simulink model "slave_site"  (R2019a)
settings: Solver=FixedStepAuto  StartTime=0.0  StopTime=inf  FixedStep=0.001  RelTol=1e-3
libraries: dspnetwork x16, etargetslib x1
settings Model: SimulationMode=accelerator  EnablePacing=on  Creator=jakub  LastModifiedBy=kirill
settings SolverCC: AutoInsertRateTranBlk=on
settings DataIOCC: ReturnWorkspaceOutputs=off
settings HardwareCC: ProdBitPerLong=64  ProdHWDeviceType=Intel->x86-64 (Linux 64)

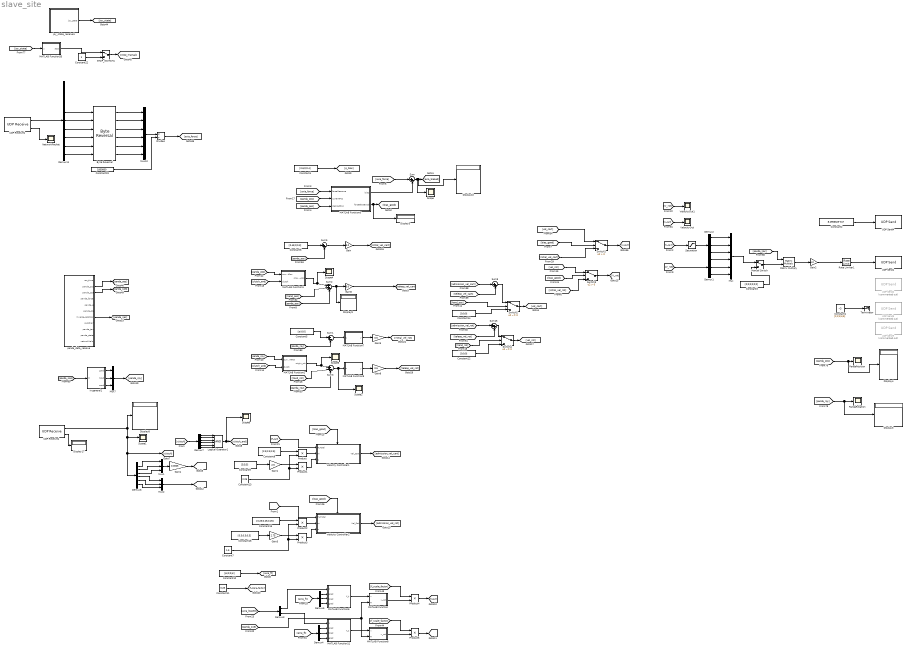
== system slave_site ==
  Byte Reversal : etargetslib/Byte Reversal  numInp=6
      settings: SourceProductName=MATLAB Coder  SourceProductBaseCode=ME
  Constant1 : Constant  Value=[1;2;3;4;5]  OutDataTypeStr=double
  Constant10 : Constant  Value=[pi/2;0;pi]
  Constant11 : Constant  Value=0.25
  Constant12 : Constant  Value=[0;0;0]
  Constant13 : Constant  Value=2.25
  Constant14 : Constant  Value=[0;0;0]
  Constant15 : Constant  Value=[0.25;0.25;0.25]
  Constant16 : Constant  Value=[0.5;0.5;0.5]
  Constant2 : Constant  Value=8.295632e-317  OutDataTypeStr=double
  Constant22 : Constant
  Constant23 : Constant  Value=1000000
  Constant3 : Constant  Value=[0;0;0;0;0;0]
  Constant4 : Constant  Value=[0.6;0;0.4]
  Constant5 : Constant  Value=[pi;0;0]
  Constant6 : Constant  Value=[0.45;0;0.3]
  Constant7 : Constant  Value=1.5
  Constant8 : Constant  Value=[2.5;2.5;2.5]
  Constant9 : Constant  Value=[5;5;5]
  Demux{1..2,4..5} (4 alike) : Demux  Outputs=3
  Demux11 : Demux  Outputs=9
  Demux3 : Demux  Outputs=2
  Demux6 : Demux  Outputs=6
  Demux7 : Demux  Outputs=6
  Display{3..5,8..10,17} (7 alike) : Display
      Display3 settings: Decimation=4
      Display4 settings: Decimation=4
  Divide4 : Product  Inputs=*/  OutDataTypeStr=double
  Gain : Gain  Gain=3.0
  Gain1 : Gain  Gain=2.5
  Gain2 : Gain  Gain=1.0
  Gain3 : Gain  Gain=2.75
  Gain4 : Gain  Gain=0.0005
  Gain5 : Gain  Gain=0.5
  Gain6 : Gain  Gain=3.0
  Gain8 : Gain  Gain=0.5
  Logical Operator1 : Logic  Inputs=6  AllPortsSameDT=off  OutDataTypeStr=boolean
  MATLAB Function : MATLAB Function  TreatAsAtomicUnit=on
  MATLAB Function1 : MATLAB Function  TreatAsAtomicUnit=on
  MATLAB Function11 : MATLAB Function  TreatAsAtomicUnit=on
  MATLAB Function2 : MATLAB Function  TreatAsAtomicUnit=on
  MATLAB Function33 : MATLAB Function  TreatAsAtomicUnit=on
  MATLAB Function5 : MATLAB Function  TreatAsAtomicUnit=on
  MATLAB Function6 : MATLAB Function  TreatAsAtomicUnit=on
  MATLAB Function7 : MATLAB Function  TreatAsAtomicUnit=on
  MATLAB Function8 : MATLAB Function  TreatAsAtomicUnit=on
  MATLAB Function9 : MATLAB Function  TreatAsAtomicUnit=on
  Manual Switch : ManualSwitch
  Matrix Multiply : Product  Multiplication=Matrix(*)
  Mux : Mux  Inputs=6
  Mux1 : Mux  Inputs=3
  Mux10 : Mux  Inputs=6
  Mux2 : Mux  Inputs=3
  Mux7 : Mux  Inputs=3
  NetworkPacket : Scope
  PandaPosition : Scope
  PandaRotation : Scope
  Product{,1..5} (6 alike) : Product
  Rate Limiter1 : RateLimiter  RisingSlewLimit=2.0  FallingSlewLimit=-2.0  SampleTimeMode=inherited
  STOP_SWITCH1 : ManualSwitch
  Saturation : Saturate  UpperLimit=0.1  LowerLimit=-0.1
  Scope{,1..2,4..6} (6 alike) : Scope
  Sum : Sum  Inputs=|+-
  Sum1 : Sum  Inputs=|+-
  Sum15 : Sum  Inputs=|++
  Sum2 : Sum  Inputs=|++-
  Sum3 : Sum  Inputs=|++-
  Sum5 : Sum  Inputs=|+-
  Sum9 : Sum  Inputs=|++
  Switch1 : Switch  Criteria=u2 > Threshold
  Switch2 : Switch  Criteria=u2 ~= 0
  Switch3 : Switch  Criteria=u2 > Threshold
  Switch4 : Switch  Criteria=u2 ~= 0
  Terminator : Terminator
  UDP Receive1 : dspnetwork/UDP Receive  localURL='0.0.0.0'  localPort=49154  remoteURL='192.168.0.13'  remotePort=-1  recvBufferSize=36  dims=9  signalDatatype=int32  isComplex=off  isVarSize=off  showBlockingTime=off  blockingTime=0  sampletime=0.001  blockPlatform=[]
      settings: SourceProductName=Simulink
  UDP Receive4 : dspnetwork/UDP Receive  localURL='0.0.0.0'  localPort=8005  remoteURL='192.168.0.110'  remotePort=-1  recvBufferSize=12288  dims=6  signalDatatype=double  isComplex=off  isVarSize=off  showBlockingTime=off  blockingTime=0  sampletime=0.001  blockPlatform=[]
      settings: SourceProductName=Simulink
  UDP Send1 : dspnetwork/UDP Send  remoteURL='127.0.0.1'  remotePort=39474  localURL='0.0.0.0'  localPortSource=Automatically determine  localPort=48000  sampletime=-1  blockPlatform=[]  separateLengthPort=0
      settings: SourceProductName=Simulink
  UDP Send2 : dspnetwork/UDP Send  Commented=on  remoteURL='255.255.255.255'  remotePort=39474  localURL='0.0.0.0'  localPortSource=Automatically determine  localPort=-1  sampletime=-1  blockPlatform=[]  separateLengthPort=0
      settings: SourceProductName=Simulink
  UDP Send3 : dspnetwork/UDP Send  Commented=on  remoteURL='192.168.0.20'  remotePort=40001  localURL='0.0.0.0'  localPortSource=Specify via dialog  localPort=49001  sampletime=-1  blockPlatform=[]  separateLengthPort=0
      settings: SourceProductName=Simulink
  UDP Send4 : dspnetwork/UDP Send  remoteURL='192.168.0.13'  remotePort=49152  localURL='0.0.0.0'  localPortSource=Specify via dialog  localPort=49154  sampletime=-1  blockPlatform=[]  separateLengthPort=0
      settings: SourceProductName=Simulink
  UDP Send5 : dspnetwork/UDP Send  Commented=on  remoteURL='127.0.0.1'  remotePort=40001  localURL='0.0.0.0'  localPortSource=Specify via dialog  localPort=49001  sampletime=-1  blockPlatform=[]  separateLengthPort=0
      settings: SourceProductName=Simulink
  Velocity Controller1 : Subsystem
  Velocity Controller2 : Subsystem
  VelocityOut : Scope
  VelocityOut1 : Scope
  in general1 : MATLAB Function  TreatAsAtomicUnit=on
  joy_state_receive1 : Subsystem
  panda_data_receive : Subsystem
  wires:
  Demux2/1 -> Mux/1
  Demux1/2 -> Mux/5
  Demux1/1 -> Mux/4
  Demux2/2 -> Mux/2
  Demux1/3 -> Mux/6
  Demux2/3 -> Mux/3
  joy_state_receive1/1("joy_state ") -> [joy_state]
  [joy_state] -> MATLAB Function33/1(u)
  MATLAB Function33/1(stop) -> STOP_SWITCH1/1
  STOP_SWITCH1/1 -> [stop_manual]
  Constant22/1 -> STOP_SWITCH1/2
  [panda_so3] -> in general1/1(R)
  in general1/2(brad) -> Mux7/2
  Mux7/1 -> [panda_rpy]
  [panda_ijac] -> Matrix Multiply/1
  UDP Receive1/2 -> NetworkPacket/1
  Byte Reversal/4 -> Mux10/4
  Divide4/1 -> [axia_force]
  Byte Reversal/2 -> Mux10/2
  Constant23/1 -> Divide4/2
  Demux11/7 -> Byte Reversal/4
  Mux10/1 -> Divide4/1
  Byte Reversal/1 -> Mux10/1
  Demux11/5 -> Byte Reversal/2
  UDP Receive1/1 -> Demux11/1
  Demux11/6 -> Byte Reversal/3
  Byte Reversal/3 -> Mux10/3
  Demux11/9 -> Byte Reversal/6
  Demux11/8 -> Byte Reversal/5
  Demux11/4 -> Byte Reversal/1
  Byte Reversal/5 -> Mux10/5
  Byte Reversal/6 -> Mux10/6
  [panda_pos] -> Display4/1, PandaPosition/1
  [V_cart] -> VelocityOut/1
  panda_data_receive/2(panda_pos) -> [panda_pos]
  panda_data_receive/3(panda_so3) -> [panda_so3]
  panda_data_receive/7(inverse_jacobian) -> [panda_ijac]
  [panda_rpy] -> Display3/1, PandaRotation/1
  [panda_rpy] -> Sum1/2
  Gain2/1 -> Rate Limiter1/1
  Matrix Multiply/1 -> Gain2/1
  Constant2/1 -> UDP Send4/1
  Constant1/1 -> Terminator/1
  Sum5/1 -> Gain/1
  [panda_pos] -> Sum5/2
  Saturation/1 -> Demux2/1
  Mux/1 -> Manual Switch/1
  Manual Switch/1 -> Matrix Multiply/2
  Constant3/1 -> Manual Switch/2
  MATLAB Function5/1(bias) -> Sum/2
  [axia_force] -> Sum/1
  Sum/1 -> Scope/1, Display10/1, [axia_biased]
  Sum1/1 -> MATLAB Function7/1(u)
  MATLAB Function7/1(y) -> Gain5/1
  MATLAB Function5/2(forceBiasGood) -> Display5/1, [bias_good]
  Constant4/1 -> [p_bias]
  [axia_force] -> MATLAB Function5/1(forceMeasure)
  [panda_pos] -> MATLAB Function5/2(currentPos)
  [panda_pos] -> MATLAB Function5/3(desiredPos)
  Constant11/1 -> [f_scale_factor]
  MATLAB Function8/1(x_rot) -> Product5/2
  MATLAB Function/1(x_rot) -> Product4/2
  Demux3/2 -> MATLAB Function11/1(X)
  Demux4/2 -> MATLAB Function11/3(brad)
  Demux5/3 -> MATLAB Function6/4(grad)
  Demux3/1 -> MATLAB Function6/1(X)
  [axia_ft] -> Demux5/1
  Demux4/3 -> MATLAB Function11/4(grad)
  Demux4/1 -> MATLAB Function11/2(arad)
  [axia_ft] -> Demux4/1
  MATLAB Function6/1(X_t) -> MATLAB Function/1(x)
  [f_scale_factor] -> Product5/1
  [f_scale_factor] -> Product4/1
  Product4/1 -> [F_cart]
  MATLAB Function11/1(X_t) -> MATLAB Function8/1(x)
  [panda_so3] -> MATLAB Function/2(R), MATLAB Function8/2(R)
  Demux5/2 -> MATLAB Function6/3(brad)
  Product5/1 -> [M_cart]
  Gain1/1 -> Product1/1
  Constant8/1 -> Product/1
  Constant9/1 -> Gain1/1
  Product/1 -> Velocity Controller1/2(m)
  Product1/1 -> Velocity Controller1/3(c)
  [F_cart] -> Velocity Controller1/1(F_Total)
  Switch1/1 -> [V_cart]
  Demux5/1 -> MATLAB Function6/2(arad)
  Constant13/1 -> Product1/2, Product/2
  [V_rot] -> VelocityOut1/1
  [axia_biased] -> Demux3/1
  Gain3/1 -> Product3/1
  Product3/1 -> Velocity Controller2/3(c)
  Constant7/1 -> Product2/2, Product3/2
  Constant16/1 -> Gain3/1
  Product2/1 -> Velocity Controller2/2(m)
  Constant15/1 -> Product2/1
  [M_cart] -> Velocity Controller2/1(M_Total)
  Switch3/1 -> [V_rot]
  [bias_good] -> Velocity Controller1/Enable
  Gain5/1 -> [initial_vel_rot]
  [initial_vel_rot] -> Switch3/3
  [bias_good] -> Velocity Controller2/Enable
  Velocity Controller2/1(Vel_Rot) -> [admission_vel_rot]
  Velocity Controller1/1(Vel_Cart) -> [admission_vel_cart]
  Gain/1 -> [initial_vel_cart]
  [initial_vel_cart] -> Switch1/3
  [vel_rot] -> Switch3/1
  [hand_pos] -> Sum2/2
  [admission_vel_cart] -> Sum9/1
  [teleop_vel_cart] -> Sum9/2
  UDP Receive4/2 -> Display17/1
  Rate Limiter1/1 -> UDP Send1/1
  [teleop_vel_rot] -> Sum15/2
  [admission_vel_rot] -> Sum15/1
  MATLAB Function9/1(y) -> Gain8/1
  [panda_rpy] -> Sum3/3
  Sum3/1 -> Scope2/1, MATLAB Function9/1(u)
  [hand_rot] -> Sum3/2
  Gain8/1 -> [teleop_vel_rot]
  UDP Receive4/1 -> Display8/1, Scope1/1, Demux6/1, [clutch]
  [vel_cart] -> Switch1/1
  Constant6/1 -> Sum5/1
  Constant10/1 -> [axia_ft]
  in general1/3(arad) -> Mux7/3
  in general1/1(grad) -> Mux7/1
  [panda_pos] -> Sum2/3
  Sum2/1 -> Gain6/1, Display9/1
  Demux6/3 -> Mux1/3
  Demux6/2 -> Mux1/2
  Demux6/1 -> Mux1/1
  Mux1/1 -> Gain4/1
  Demux6/4 -> Mux2/1
  Demux6/5 -> Mux2/2
  Demux6/6 -> Mux2/3
  [bias_good] -> Switch1/2
  [panda_pos] -> MATLAB Function1/1(currentPos)
  MATLAB Function1/1(origin_pos) -> Scope4/1, Sum2/1
  [clutch_and] -> MATLAB Function1/2(clutch)
  Demux7/1 -> Logical Operator1/1
  Demux7/2 -> Logical Operator1/2
  Demux7/6 -> Logical Operator1/6
  Demux7/3 -> Logical Operator1/3
  Demux7/4 -> Logical Operator1/4
  [clutch] -> Demux7/1
  Demux7/5 -> Logical Operator1/5
  Logical Operator1/1 -> Scope6/1, [clutch_and]
  Gain4/1 -> [hand_pos]
  Mux2/1 -> [hand_rot]
  Constant5/1 -> Sum1/1
  [bias_good] -> Switch3/2
  [clutch_and] -> MATLAB Function2/2(clutch)
  [panda_rpy] -> MATLAB Function2/1(currentRot)
  MATLAB Function2/1(origin_rot) -> Scope5/1, Sum3/1
  Switch2/1 -> [vel_cart]
  Sum9/1 -> Switch2/1
  Constant14/1 -> Switch2/3
  [hand_pos] -> Switch2/2
  Switch4/1 -> [vel_rot]
  Sum15/1 -> Switch4/1
  Constant12/1 -> Switch4/3
  [hand_rot] -> Switch4/2
  Gain6/1 -> [teleop_vel_cart]
  [V_cart] -> Saturation/1
  [V_rot] -> Demux1/1

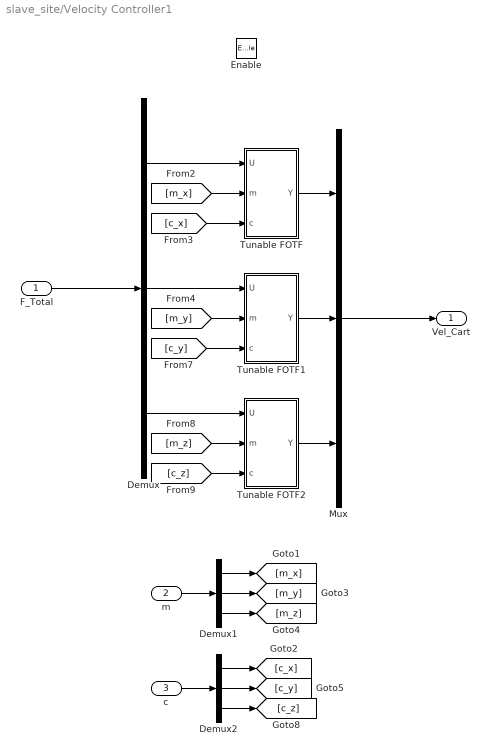
== system slave_site/Velocity Controller1 ==
  F_Total : Inport
  m : Inport  Port=2
  c : Inport  Port=3
  Enable : EnablePort
  Demux : Demux  Outputs=3
  Demux1 : Demux  Outputs=3
  Demux2 : Demux  Outputs=3
  Mux : Mux  Inputs=3
  Tunable FOTF : Subsystem
  Tunable FOTF1 : Subsystem
  Tunable FOTF2 : Subsystem
  Vel_Cart : Outport
  wires:
  [m_y] -> Tunable FOTF1/2(m)
  [c_x] -> Tunable FOTF/3(c)
  Demux/1 -> Tunable FOTF/1(U)
  Tunable FOTF2/1(Y) -> Mux/3
  [m_z] -> Tunable FOTF2/2(m)
  Mux/1 -> Vel_Cart/1
  [c_y] -> Tunable FOTF1/3(c)
  [m_x] -> Tunable FOTF/2(m)
  [c_z] -> Tunable FOTF2/3(c)
  Tunable FOTF/1(Y) -> Mux/1
  Demux/2 -> Tunable FOTF1/1(U)
  F_Total/1 -> Demux/1
  Tunable FOTF1/1(Y) -> Mux/2
  Demux/3 -> Tunable FOTF2/1(U)
  Demux2/2 -> [c_y]
  Demux1/2 -> [m_y]
  c/1 -> Demux2/1
  m/1 -> Demux1/1
  Demux2/1 -> [c_x]
  Demux1/1 -> [m_x]
  Demux1/3 -> [m_z]
  Demux2/3 -> [c_z]

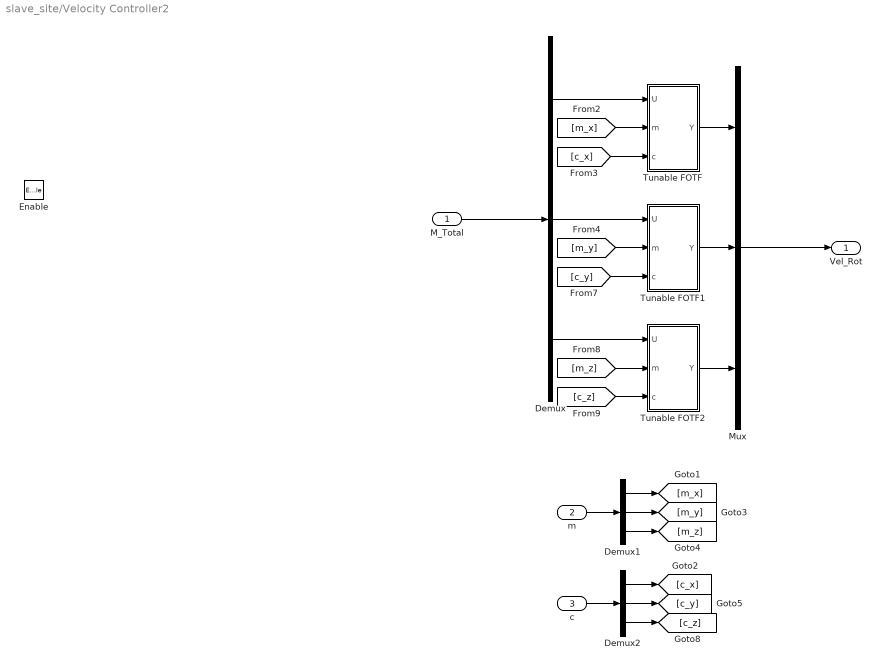
== system slave_site/Velocity Controller2 ==
  M_Total : Inport
  m : Inport  Port=2
  c : Inport  Port=3
  Enable : EnablePort
  Demux : Demux  Outputs=3
  Demux1 : Demux  Outputs=3
  Demux2 : Demux  Outputs=3
  Mux : Mux  Inputs=3
  Tunable FOTF : Subsystem
  Tunable FOTF1 : Subsystem
  Tunable FOTF2 : Subsystem
  Vel_Rot : Outport
  wires:
  [m_y] -> Tunable FOTF1/2(m)
  [c_x] -> Tunable FOTF/3(c)
  Demux/1 -> Tunable FOTF/1(U)
  Tunable FOTF2/1(Y) -> Mux/3
  [m_z] -> Tunable FOTF2/2(m)
  Mux/1 -> Vel_Rot/1
  [c_y] -> Tunable FOTF1/3(c)
  [m_x] -> Tunable FOTF/2(m)
  [c_z] -> Tunable FOTF2/3(c)
  Tunable FOTF/1(Y) -> Mux/1
  Demux/2 -> Tunable FOTF1/1(U)
  M_Total/1 -> Demux/1
  Tunable FOTF1/1(Y) -> Mux/2
  Demux/3 -> Tunable FOTF2/1(U)
  Demux2/2 -> [c_y]
  Demux1/2 -> [m_y]
  c/1 -> Demux2/1
  m/1 -> Demux1/1
  Demux2/1 -> [c_x]
  Demux1/1 -> [m_x]
  Demux1/3 -> [m_z]
  Demux2/3 -> [c_z]

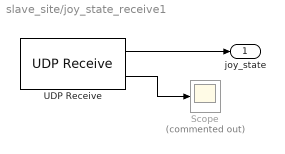
== system slave_site/joy_state_receive1 ==
  Scope : Scope  Commented=on
  UDP Receive : dspnetwork/UDP Receive  localURL='0.0.0.0'  localPort=33333  remoteURL='0.0.0.0'  remotePort=-1  recvBufferSize=840  dims=21  signalDatatype=single  isComplex=off  isVarSize=off  showBlockingTime=off  blockingTime=0  sampletime=0.001  blockPlatform=[]
      settings: SourceProductName=Simulink
  "joy_state " : Outport
  wires:
  UDP Receive/2 -> Scope/1
  UDP Receive/1 -> "joy_state "/1

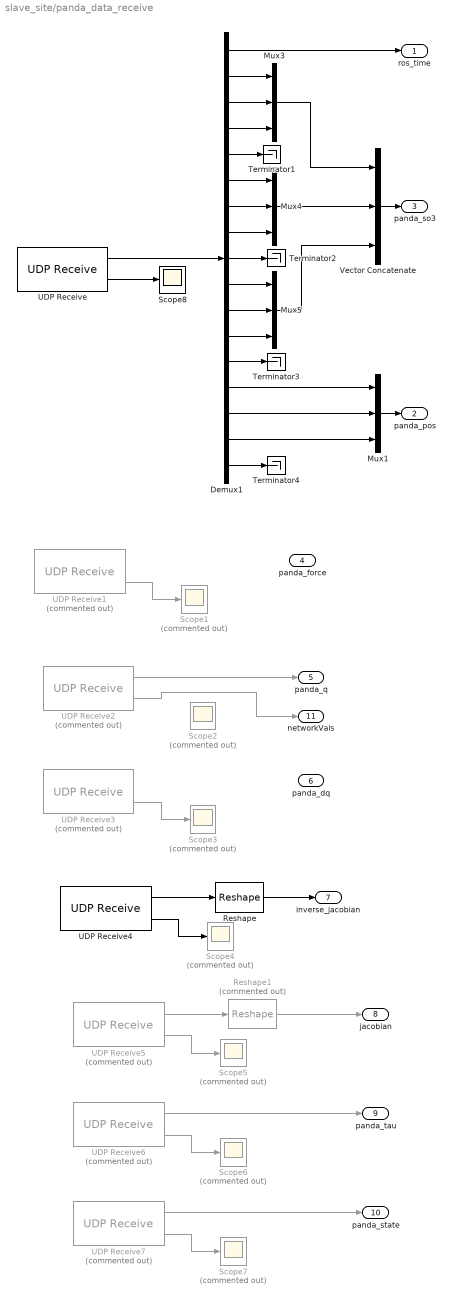
== system slave_site/panda_data_receive ==
  Demux1 : Demux  Outputs=17
  Mux{1,3..5} (4 alike) : Mux  Inputs=3
  Reshape : Reshape  OutputDimensionality=Customize  OutputDimensions=[7,6]
  Reshape1 : Reshape  Commented=on  OutputDimensionality=Customize  OutputDimensions=[7,6]
  Scope{1..7} (7 alike) : Scope  Commented=on
  Scope8 : Scope
  Terminator{1..4} (4 alike) : Terminator
  UDP Receive : dspnetwork/UDP Receive  localURL='0.0.0.0'  localPort=30001  remoteURL='127.0.0.1'  remotePort=-1  recvBufferSize=4096  dims=17  signalDatatype=double  isComplex=off  isVarSize=off  showBlockingTime=off  blockingTime=0  sampletime=0.001  blockPlatform=[]
      settings: SourceProductName=Simulink
  UDP Receive1 : dspnetwork/UDP Receive  Commented=on  localURL='0.0.0.0'  localPort=30002  remoteURL='0.0.0.0'  remotePort=-1  recvBufferSize=48  dims=6  signalDatatype=double  isComplex=off  isVarSize=off  showBlockingTime=off  blockingTime=0  sampletime=0.001  blockPlatform=[]
      settings: SourceProductName=Simulink
  UDP Receive2 : dspnetwork/UDP Receive  Commented=on  localURL='0.0.0.0'  localPort=30003  remoteURL='0.0.0.0'  remotePort=-1  recvBufferSize=56  dims=7  signalDatatype=double  isComplex=off  isVarSize=off  showBlockingTime=off  blockingTime=0  sampletime=0.001  blockPlatform=[]
      settings: SourceProductName=Simulink
  UDP Receive3 : dspnetwork/UDP Receive  Commented=on  localURL='0.0.0.0'  localPort=30004  remoteURL='0.0.0.0'  remotePort=-1  recvBufferSize=56  dims=7  signalDatatype=double  isComplex=off  isVarSize=off  showBlockingTime=off  blockingTime=0  sampletime=0.001  blockPlatform=[]
      settings: SourceProductName=Simulink
  UDP Receive4 : dspnetwork/UDP Receive  localURL='0.0.0.0'  localPort=30005  remoteURL='0.0.0.0'  remotePort=-1  recvBufferSize=3360  dims=42  signalDatatype=double  isComplex=off  isVarSize=off  showBlockingTime=off  blockingTime=0  sampletime=0.001  blockPlatform=[]
      settings: SourceProductName=Simulink
  UDP Receive5 : dspnetwork/UDP Receive  Commented=on  localURL='0.0.0.0'  localPort=30006  remoteURL='0.0.0.0'  remotePort=-1  recvBufferSize=3360  dims=42  signalDatatype=double  isComplex=off  isVarSize=off  showBlockingTime=off  blockingTime=0  sampletime=0.001  blockPlatform=[]
      settings: SourceProductName=Simulink
  UDP Receive6 : dspnetwork/UDP Receive  Commented=on  localURL='0.0.0.0'  localPort=30010  remoteURL='0.0.0.0'  remotePort=-1  recvBufferSize=56  dims=7  signalDatatype=double  isComplex=off  isVarSize=off  showBlockingTime=off  blockingTime=0  sampletime=0.001  blockPlatform=[]
      settings: SourceProductName=Simulink
  UDP Receive7 : dspnetwork/UDP Receive  Commented=on  localURL='0.0.0.0'  localPort=30030  remoteURL='0.0.0.0'  remotePort=-1  recvBufferSize=40  dims=1  signalDatatype=uint8  isComplex=off  isVarSize=off  showBlockingTime=off  blockingTime=0  sampletime=0.001  blockPlatform=[]
      settings: SourceProductName=Simulink
  Vector Concatenate : Concatenate  NumInputs=3  Mode=Multidimensional array  ConcatenateDimension=2
  ros_time : Outport
  panda_pos : Outport  Port=2
  panda_so3 : Outport  Port=3
  panda_force : Outport  Port=4
  panda_q : Outport  Port=5
  panda_dq : Outport  Port=6
  inverse_jacobian : Outport  Port=7
  jacobian : Outport  Port=8
  panda_tau : Outport  Port=9
  panda_state : Outport  Port=10
  networkVals : Outport  Port=11
  wires:
  Mux1/1 -> panda_pos/1
  Demux1/6 -> Mux4/1
  Mux3/1 -> Vector Concatenate/1
  Demux1/10 -> Mux5/1
  Demux1/7 -> Mux4/2
  Demux1/12 -> Mux5/3
  Demux1/16 -> Mux1/3
  Demux1/9 -> Terminator2/1
  Demux1/4 -> Mux3/3
  Demux1/15 -> Mux1/2
  Demux1/5 -> Terminator1/1
  Demux1/2 -> Mux3/1
  Demux1/3 -> Mux3/2
  Demux1/1 -> ros_time/1
  Demux1/14 -> Mux1/1
  Mux4/1 -> Vector Concatenate/2
  Demux1/8 -> Mux4/3
  Demux1/11 -> Mux5/2
  Vector Concatenate/1 -> panda_so3/1
  Demux1/13 -> Terminator3/1
  Demux1/17 -> Terminator4/1
  Mux5/1 -> Vector Concatenate/3
  UDP Receive1/2 -> Scope1/1
  UDP Receive2/1 -> panda_q/1
  UDP Receive3/2 -> Scope3/1
  Reshape/1 -> inverse_jacobian/1
  UDP Receive4/2 -> Scope4/1
  UDP Receive4/1 -> Reshape/1
  Reshape1/1 -> jacobian/1
  UDP Receive5/1 -> Reshape1/1
  UDP Receive5/2 -> Scope5/1
  UDP Receive6/1 -> panda_tau/1
  UDP Receive6/2 -> Scope6/1
  UDP Receive7/1 -> panda_state/1
  UDP Receive7/2 -> Scope7/1
  UDP Receive2/2 -> networkVals/1
  UDP Receive/2 -> Scope8/1
  UDP Receive/1 -> Demux1/1

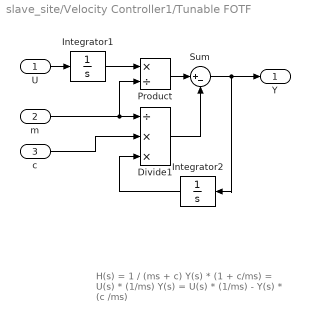
== system slave_site/Velocity Controller1/Tunable FOTF ==
  note: H(s) = 1 / (ms + c)
      | Y(s) * (1 + c/ms) = U(s) * (1/ms)
      | Y(s) = U(s) * (1/ms) - Y(s) * (c /ms)
  U : Inport
  m : Inport  Port=2
  c : Inport  Port=3
  Divide1 : Product  Inputs=/**
  Integrator1 : Integrator
  Integrator2 : Integrator
  Product : Product  Inputs=*/
  Sum : Sum  Inputs=|+-
  Y : Outport
  wires:
  U/1 -> Integrator1/1
  Integrator1/1 -> Product/1
  m/1 -> Divide1/1, Product/2
  Product/1 -> Sum/1
  Sum/1 -> Integrator2/1, Y/1
  c/1 -> Divide1/2
  Divide1/1 -> Sum/2
  Integrator2/1 -> Divide1/3

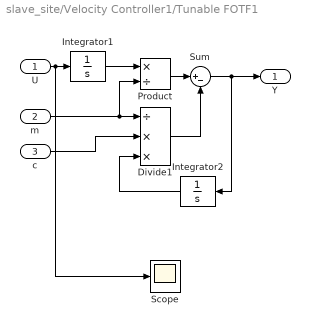
== system slave_site/Velocity Controller1/Tunable FOTF1 ==
  U : Inport
  m : Inport  Port=2
  c : Inport  Port=3
  Divide1 : Product  Inputs=/**
  Integrator1 : Integrator
  Integrator2 : Integrator
  Product : Product  Inputs=*/
  Scope : Scope
  Sum : Sum  Inputs=|+-
  Y : Outport
  wires:
  U/1 -> Scope/1, Integrator1/1
  Integrator1/1 -> Product/1
  m/1 -> Divide1/1, Product/2
  Product/1 -> Sum/1
  Sum/1 -> Integrator2/1, Y/1
  c/1 -> Divide1/2
  Divide1/1 -> Sum/2
  Integrator2/1 -> Divide1/3

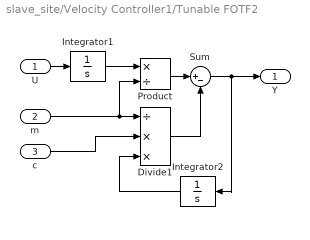
== system slave_site/Velocity Controller1/Tunable FOTF2 ==
  U : Inport
  m : Inport  Port=2
  c : Inport  Port=3
  Divide1 : Product  Inputs=/**
  Integrator1 : Integrator
  Integrator2 : Integrator
  Product : Product  Inputs=*/
  Sum : Sum  Inputs=|+-
  Y : Outport
  wires:
  U/1 -> Integrator1/1
  Integrator1/1 -> Product/1
  m/1 -> Divide1/1, Product/2
  Product/1 -> Sum/1
  Sum/1 -> Integrator2/1, Y/1
  c/1 -> Divide1/2
  Divide1/1 -> Sum/2
  Integrator2/1 -> Divide1/3

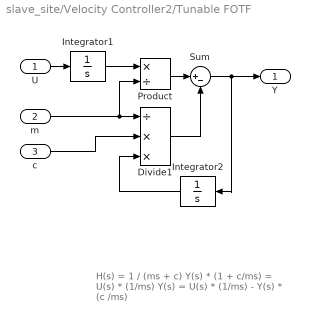
== system slave_site/Velocity Controller2/Tunable FOTF ==
  note: H(s) = 1 / (ms + c)
      | Y(s) * (1 + c/ms) = U(s) * (1/ms)
      | Y(s) = U(s) * (1/ms) - Y(s) * (c /ms)
  U : Inport
  m : Inport  Port=2
  c : Inport  Port=3
  Divide1 : Product  Inputs=/**
  Integrator1 : Integrator
  Integrator2 : Integrator
  Product : Product  Inputs=*/
  Sum : Sum  Inputs=|+-
  Y : Outport
  wires:
  U/1 -> Integrator1/1
  Integrator1/1 -> Product/1
  m/1 -> Divide1/1, Product/2
  Product/1 -> Sum/1
  Sum/1 -> Integrator2/1, Y/1
  c/1 -> Divide1/2
  Divide1/1 -> Sum/2
  Integrator2/1 -> Divide1/3

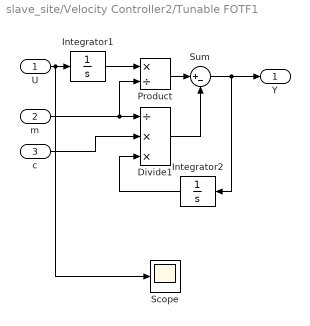
== system slave_site/Velocity Controller2/Tunable FOTF1 ==
  U : Inport
  m : Inport  Port=2
  c : Inport  Port=3
  Divide1 : Product  Inputs=/**
  Integrator1 : Integrator
  Integrator2 : Integrator
  Product : Product  Inputs=*/
  Scope : Scope
  Sum : Sum  Inputs=|+-
  Y : Outport
  wires:
  U/1 -> Scope/1, Integrator1/1
  Integrator1/1 -> Product/1
  m/1 -> Divide1/1, Product/2
  Product/1 -> Sum/1
  Sum/1 -> Integrator2/1, Y/1
  c/1 -> Divide1/2
  Divide1/1 -> Sum/2
  Integrator2/1 -> Divide1/3

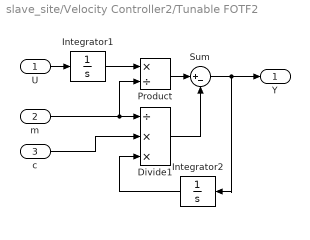
== system slave_site/Velocity Controller2/Tunable FOTF2 ==
  U : Inport
  m : Inport  Port=2
  c : Inport  Port=3
  Divide1 : Product  Inputs=/**
  Integrator1 : Integrator
  Integrator2 : Integrator
  Product : Product  Inputs=*/
  Sum : Sum  Inputs=|+-
  Y : Outport
  wires:
  U/1 -> Integrator1/1
  Integrator1/1 -> Product/1
  m/1 -> Divide1/1, Product/2
  Product/1 -> Sum/1
  Sum/1 -> Integrator2/1, Y/1
  c/1 -> Divide1/2
  Divide1/1 -> Sum/2
  Integrator2/1 -> Divide1/3

== matlab function slave_site/MATLAB Function2 ==
  data: currentRot input; origin_rot output; clutch input
function origin_rot = fcn(currentRot, clutch)
    persistent originRot
    
    if isempty(originRot)
        originRot = currentRot;
    end
    
    if clutch == 0
        originRot = currentRot;
    end

    
origin_rot = originRot;


end

== matlab function slave_site/MATLAB Function1 ==
  data: currentPos input; origin_pos output; clutch input
function origin_pos = fcn(currentPos, clutch)
    persistent originPos
    
    if isempty(originPos)
        originPos = currentPos;
    end
    
    if clutch == 0
        originPos = currentPos;
    end

    
origin_pos = originPos;


end

== matlab function slave_site/MATLAB Function ==
  data: x input; x_rot output; R input
function x_rot = rot(x,R)
%#codegen
x_rot = R*x;
end

== matlab function slave_site/MATLAB Function5 ==
  data: forceMeasure input; bias output; forceBiasGood output; currentPos input; desiredPos input
function [bias, forceBiasGood] = forceBias(forceMeasure,currentPos,desiredPos)
    persistent n force_sensor_data
    data_limit = 5000;
    pos_max_error = 0.0007;
    
    if isempty(force_sensor_data)    
        force_sensor_data = zeros(6,data_limit);
    end
    
    if isempty(n)
        n = 1;
    end
    
    errPos = sum(abs(currentPos - desiredPos));
    if(errPos <= pos_max_error && n <= data_limit)
    %if(n <= data_limit && biasPosGood)
        if(sum(abs(forceMeasure)) ~= 0)
            force_sensor_data(:,n) = forceMeasure;
            n = n + 1;
        end
    end
    
    bias = zeros(6,1);
    forceBiasGood = false;
    
    if(n > data_limit)
        force_sensor_data_means = mean(force_sensor_data,2);
        bias(:) = force_sensor_data_means;
        forceBiasGood = true;
    end

== matlab function slave_site/MATLAB Function11 ==
  data: X input; X_t output; arad input; brad input; grad input
function X_t  = rot(X,arad,brad,grad)
%#codegen
Rz = [cos(arad) -sin(arad) 0; sin(arad) cos(arad) 0; 0 0 1];
Ry = [cos(brad) 0 sin(brad); 0 1 0; -sin(brad) 0 cos(brad)];
Rx = [1 0 0; 0 cos(grad) -sin(grad); 0 sin(grad) cos(grad)];
T = Rz * Ry * Rx;
T = -T;
X_t = T*X;

== matlab function slave_site/MATLAB Function7 ==
  data: u input; y output
function y = fcn(u)
    for i = 1:3
        if u(i)>pi
            u(i) = u(i)-(2*pi)
        elseif u(i)<-pi
            u(i) = u(i)+(2*pi)
        end
    end
y = u;

== matlab function slave_site/MATLAB Function6 ==
  data: X input; X_t output; arad input; brad input; grad input
function X_t  = rot(X,arad,brad,grad)
%#codegen
Rz = [cos(arad) -sin(arad) 0; sin(arad) cos(arad) 0; 0 0 1];
Ry = [cos(brad) 0 sin(brad); 0 1 0; -sin(brad) 0 cos(brad)];
Rx = [1 0 0; 0 cos(grad) -sin(grad); 0 sin(grad) cos(grad)];
T = Rz * Ry * Rx;
T = -T;
X_t = T*X;

== matlab function slave_site/MATLAB Function8 ==
  data: x input; x_rot output; R input
function x_rot = rot(x,R)
%#codegen
x_rot = R*x;
end

== matlab function slave_site/MATLAB Function9 ==
  data: u input; y output
function y = fcn(u)
    for i = 1:3
        if u(i)>pi
            u(i) = u(i)-(2*pi)
        elseif u(i)<-pi
            u(i) = u(i)+(2*pi)
        end
    end
y = u;

== matlab function slave_site/in general1 ==
  data: grad output; brad output; arad output; R input
function [grad,brad,arad] = so3_to_rpy(R)
sy = sqrt(R(3,2)^2 + R(3,3)^2);
if sy > eps
    % non singular
    grad = atan2(R(3,2),R(3,3));
    brad = atan2(-R(3,1),sy);
    arad = atan2(R(2,1),R(1,1));
else
    % singular
    grad = atan2(-R(2,3),R(2,2));
    brad = atan2(-R(3,1),sy);
    arad = 0;
end
end

== matlab function slave_site/MATLAB Function33 ==
  data: u input; stop output
function stop = fcn(u)
if u(16) == 1 && u(17) == 1
    stop = 1;
else
    stop = 0;
end
